simulink model "Assignment2_2017"  (R2017b)
settings: Solver=FixedStepAuto  StartTime=0.0  StopTime=inf  FixedStep=1E-3  RelTol=1e-3  EnableMultiTasking=on
undefined symbols (not defined in the file): D0, D1, D10, D11, D12, D13, D2, D5, D8, D9, PTA0, PTA2, PTB9, PTC16, PTC17, PTC4, PTD0, PTD1, PTD2, PTD3
libraries: frdmk64flib x13, dspswit3 x2
settings Model: ExtModeTrigDuration=5  Creator=Hassan  LastModifiedBy=Hassan
settings OptimizationCC: EnhancedBackFolding=on  PassReuseOutputArgsAs=Individual arguments  MaxStackSize=64  OptimizeBlockOrder=speed  DifferentSizesBufferReuse=on
settings DebuggingCC: ParameterTunabilityLossMsg=error
settings HardwareCC: ProdBitPerPointer=32  ProdBitPerSizeT=32  ProdBitPerPtrDiffT=32  ProdLargestAtomicInteger=Long  ProdLargestAtomicFloat=Double  ProdWordSize=32  ProdHWDeviceType=ARM Compatible->ARM Cortex  UseEmbeddedCoderFeatures=off
settings SFSimCC: SimUseLocalCustomCode=on  MATLABDynamicMemAlloc=off
settings RTWCC: SystemTargetFile=ert.tlc  HardwareBoard=NXP FRDM-K64F  TemplateMakefile=ert_default_tmf  GenerateReport=on  RTWUseLocalCustomCode=on  Toolchain=GNU Tools for ARM Embedded Processors  IncludeHyperlinkInReport=on  LaunchReport=on  GenerateTraceInfo=on  GenerateTraceReport=on  GenerateTraceReportSl=on  GenerateTraceReportSf=on  GenerateTraceReportEml=on
settings CodeAppCC: ForceParamTrailComments=on  IgnoreCustomStorageClasses=off  OperatorAnnotations=on  SimulinkDataObjDesc=on  SFDataObjDesc=on  InsertBlockDesc=on
settings ERTTargetCC: SupportNonInlinedSFcns=on

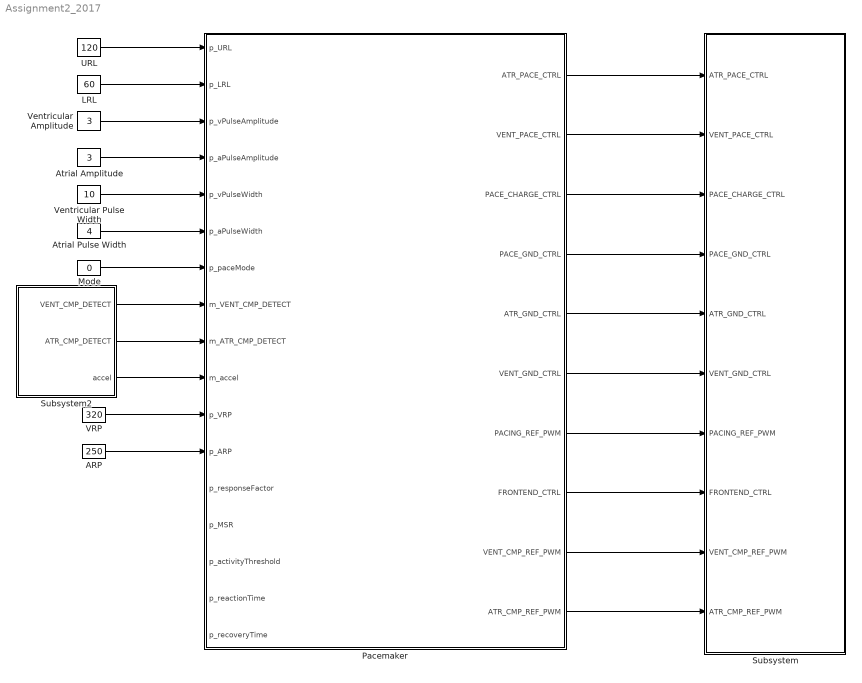
== system Assignment2_2017 ==
  ARP : Constant  Value=250  OutDataTypeStr=double
  Atrial Amplitude : Constant  Value=3  OutDataTypeStr=double
  Atrial Pulse Width : Constant  Value=4  OutDataTypeStr=double
  LRL : Constant  Value=60  OutDataTypeStr=double
  Mode : Constant  Value=0  OutDataTypeStr=uint8
  Pacemaker : Stateflow chart  TreatAsAtomicUnit=on
  Subsystem : Subsystem
  Subsystem2 : Subsystem
  URL : Constant  Value=120  OutDataTypeStr=double
  VRP : Constant  Value=320  OutDataTypeStr=double
  Ventricular Amplitude : Constant  Value=3  OutDataTypeStr=double
  Ventricular Pulse Width : Constant  Value=10  OutDataTypeStr=double
  wires:
  Ventricular Pulse Width/1 -> Pacemaker/5(p_vPulseWidth)
  Mode/1 -> Pacemaker/7(p_paceMode)
  Atrial Pulse Width/1 -> Pacemaker/6(p_aPulseWidth)
  Ventricular Amplitude/1 -> Pacemaker/3(p_vPulseAmplitude)
  LRL/1 -> Pacemaker/2(p_LRL)
  URL/1 -> Pacemaker/1(p_URL)
  Atrial Amplitude/1 -> Pacemaker/4(p_aPulseAmplitude)
  Pacemaker/1(ATR_PACE_CTRL) -> Subsystem/1(ATR_PACE_CTRL)
  Pacemaker/2(VENT_PACE_CTRL) -> Subsystem/2(VENT_PACE_CTRL)
  Pacemaker/3(PACE_CHARGE_CTRL) -> Subsystem/3(PACE_CHARGE_CTRL)
  Pacemaker/4(PACE_GND_CTRL) -> Subsystem/4(PACE_GND_CTRL)
  Pacemaker/5(ATR_GND_CTRL) -> Subsystem/5(ATR_GND_CTRL)
  Pacemaker/6(VENT_GND_CTRL) -> Subsystem/6(VENT_GND_CTRL)
  Pacemaker/7(PACING_REF_PWM) -> Subsystem/7(PACING_REF_PWM)
  Pacemaker/9(VENT_CMP_REF_PWM) -> Subsystem/9(VENT_CMP_REF_PWM)
  Pacemaker/8(FRONTEND_CTRL) -> Subsystem/8(FRONTEND_CTRL)
  Pacemaker/10(ATR_CMP_REF_PWM) -> Subsystem/10(ATR_CMP_REF_PWM)
  VRP/1 -> Pacemaker/11(p_VRP)
  ARP/1 -> Pacemaker/12(p_ARP)
  Subsystem2/1(VENT_CMP_DETECT) -> Pacemaker/8(m_VENT_CMP_DETECT)
  Subsystem2/2(ATR_CMP_DETECT) -> Pacemaker/9(m_ATR_CMP_DETECT)
  Subsystem2/3(accel) -> Pacemaker/10(m_accel)

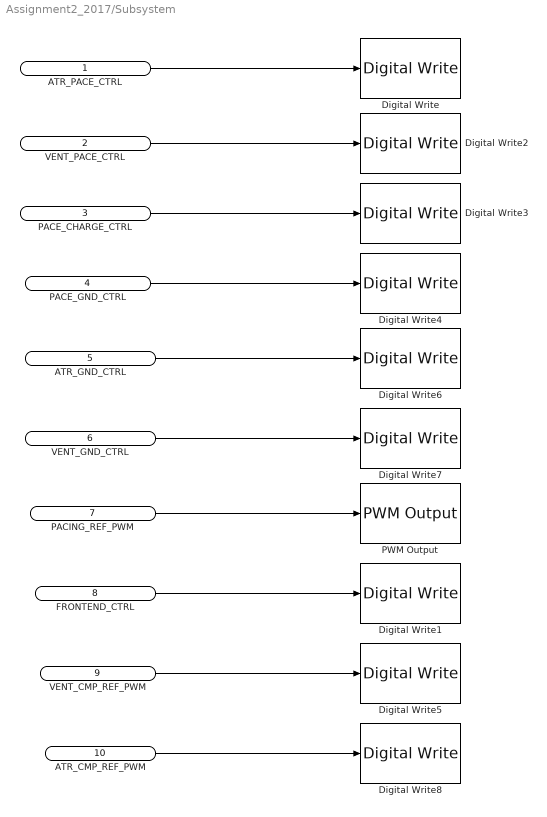
== system Assignment2_2017/Subsystem ==
  ATR_PACE_CTRL : Inport
  VENT_PACE_CTRL : Inport  Port=2
  PACE_CHARGE_CTRL : Inport  Port=3
  PACE_GND_CTRL : Inport  Port=4
  ATR_GND_CTRL : Inport  Port=5
  VENT_GND_CTRL : Inport  Port=6
  PACING_REF_PWM : Inport  Port=7
  FRONTEND_CTRL : Inport  Port=8
  VENT_CMP_REF_PWM : Inport  Port=9
  ATR_CMP_REF_PWM : Inport  Port=10
  Digital Write : frdmk64flib/Digital Write  Whichpin=PTA0 (D8)
      settings: SourceProductName=Simulink Coder Support Package for NXP FRDM-K64F Board
  Digital Write1 : frdmk64flib/Digital Write  Whichpin=PTD1 (D13)
      settings: SourceProductName=Simulink Coder Support Package for NXP FRDM-K64F Board
  Digital Write2 : frdmk64flib/Digital Write  Whichpin=PTC4 (D9)
      settings: SourceProductName=Simulink Coder Support Package for NXP FRDM-K64F Board
  Digital Write3 : frdmk64flib/Digital Write  Whichpin=PTB9 (D2)
      settings: SourceProductName=Simulink Coder Support Package for NXP FRDM-K64F Board
  Digital Write4 : frdmk64flib/Digital Write  Whichpin=PTD0 (D10)
      settings: SourceProductName=Simulink Coder Support Package for NXP FRDM-K64F Board
  Digital Write5 : frdmk64flib/Digital Write  Whichpin=RED_LED
      settings: SourceProductName=Simulink Coder Support Package for NXP FRDM-K64F Board
  Digital Write6 : frdmk64flib/Digital Write  Whichpin=PTD2 (D11)
      settings: SourceProductName=Simulink Coder Support Package for NXP FRDM-K64F Board
  Digital Write7 : frdmk64flib/Digital Write  Whichpin=PTD3 (D12)
      settings: SourceProductName=Simulink Coder Support Package for NXP FRDM-K64F Board
  Digital Write8 : frdmk64flib/Digital Write  Whichpin=RED_LED
      settings: SourceProductName=Simulink Coder Support Package for NXP FRDM-K64F Board
  PWM Output : frdmk64flib/PWM Output  Whichpin=PTA2 (D5)  InitialFrequency=1000  InitialDutyCycle=0
      settings: SourceProductName=Simulink Coder Support Package for NXP FRDM-K64F Board
  wires:
  ATR_PACE_CTRL/1 -> Digital Write/1
  VENT_PACE_CTRL/1 -> Digital Write2/1
  PACE_CHARGE_CTRL/1 -> Digital Write3/1
  PACE_GND_CTRL/1 -> Digital Write4/1
  ATR_GND_CTRL/1 -> Digital Write6/1
  VENT_GND_CTRL/1 -> Digital Write7/1
  PACING_REF_PWM/1 -> PWM Output/1
  FRONTEND_CTRL/1 -> Digital Write1/1
  ATR_CMP_REF_PWM/1 -> Digital Write8/1
  VENT_CMP_REF_PWM/1 -> Digital Write5/1

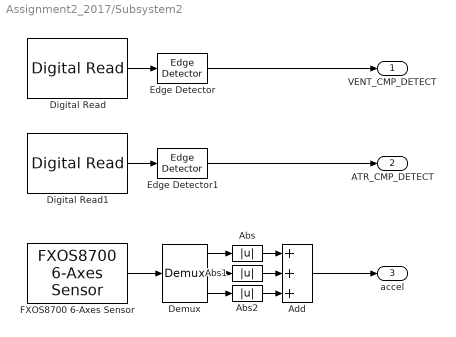
== system Assignment2_2017/Subsystem2 ==
  Abs : Abs
  Abs1 : Abs
  Abs2 : Abs
  Add : Sum  Inputs=+++
  Demux : Demux  Outputs=3
  Digital Read : frdmk64flib/Digital Read  Whichpin=PTC17 (D1)  SampleTime=-1
      settings: SourceProductName=Simulink Coder Support Package for NXP FRDM-K64F Board
  Digital Read1 : frdmk64flib/Digital Read  Whichpin=PTC16 (D0)  SampleTime=-1
      settings: SourceProductName=Simulink Coder Support Package for NXP FRDM-K64F Board
  Edge Detector : dspswit3/Edge Detector
      settings: SourceProductName=DSP System Toolbox  SourceProductBaseCode=DS
  Edge Detector1 : dspswit3/Edge Detector
      settings: SourceProductName=DSP System Toolbox  SourceProductBaseCode=DS
  FXOS8700 6-Axes Sensor : frdmk64flib/FXOS8700 6-Axes Sensor  Activesensor=Accelerometer only  ODR=400Hz  HybridODR=400Hz  Accelfullrange=-4g to +4g  SampleTime=-1
      settings: SourceProductName=Simulink Coder Support Package for NXP FRDM-K64F Board
  VENT_CMP_DETECT : Outport
  ATR_CMP_DETECT : Outport  Port=2
  accel : Outport  Port=3
  wires:
  Digital Read/1 -> Edge Detector/1
  Digital Read1/1 -> Edge Detector1/1
  Edge Detector1/1 -> ATR_CMP_DETECT/1
  Edge Detector/1 -> VENT_CMP_DETECT/1
  FXOS8700 6-Axes Sensor/1 -> Demux/1
  Add/1 -> accel/1
  Demux/1 -> Abs/1
  Abs/1 -> Add/1
  Demux/2 -> Abs1/1
  Abs1/1 -> Add/2
  Demux/3 -> Abs2/1
  Abs2/1 -> Add/3

== stateflow chart Assignment2_2017/Pacemaker ==
  state Init
  state SetPulseRate
    entry:
    VVtime=(60000/p_LRL)-p_vPulseWidth;
    AAtime=(60000/p_LRL)-p_aPulseWidth;
  state VentricleSensingInit
    entry:
    VENT_CMP_REF_PWM = (3.3/3.3)*100;
    FRONTEND_CTRL=1;
  state ModeChange
    entry:
    FRONTEND_CTRL=0;
  state AtriumSensingInit
    entry:
    ATR_CMP_REF_PWM = (3.3/3.3)*100;
    FRONTEND_CTRL=1;
  state ChargeC22DischargeC21
    % Charging C22 and discharging C21
    entry:
    % Charge C22
    VENT_PACE_CTRL=0;
    PACING_REF_PWM=(pulseAmplitude/5.0)*100;
    PACE_CHARGE_CTRL=1;
    %Discharge C21
    PACE_GND_CTRL=1;
    VENT_GND_CTRL=1;
  state PaceAtrium
    %PACE ATRIUM
    entry:
    PACE_CHARGE_CTRL=0;
    PACE_GND_CTRL=1;
    ATR_GND_CTRL=0;
    ATR_PACE_CTRL=1;
  state CheckAccelUpdateRate
    entry:
    updateRate();
  state PaceVentricle
    %PACE VENTRICLE
    entry:
    PACE_CHARGE_CTRL=0;
    PACE_GND_CTRL=1;
    VENT_GND_CTRL=0;
    VENT_PACE_CTRL=1;
  state VRP
  state ARP
  state VentBeatSensed
  state AtrBeatSensed
  (default) -> Init
  Init -> SetPulseRate
  (junction 72) -> VentricleSensingInit [order 1] : [p_paceMode==4 || p_paceMode==5]
  SetPulseRate -> (junction 72) [order 1] : [p_paceMode>=4]
  ModeChange -> SetPulseRate
  (junction 72) -> AtriumSensingInit [order 2] : [p_paceMode==6 || p_paceMode==7]
  VentricleSensingInit -> (junction 84)
  SetPulseRate -> ChargeC22DischargeC21 [order 2] : [p_paceMode<4]
  AtriumSensingInit -> (junction 84)
  (junction 84) -> ChargeC22DischargeC21
  (junction 144) -> ModeChange [order 2]
  ChargeC22DischargeC21 -> PaceAtrium [order 4] : [(p_paceMode==2 || p_paceMode==3) && after(AAtime, msec)]
  PaceAtrium -> (junction 144) : [after(p_aPulseWidth,msec)]
  CheckAccelUpdateRate -> ModeChange
  PaceVentricle -> (junction 144) : [after(p_vPulseWidth,msec)]
  (junction 144) -> CheckAccelUpdateRate [order 1] : [p_paceMode==1 || p_paceMode==3]
  ChargeC22DischargeC21 -> PaceVentricle [order 3] : [(p_paceMode==0 || p_paceMode==1) && after(VVtime, msec)]
  ChargeC22DischargeC21 -> VentBeatSensed [order 2] : [m_VENT_CMP_DETECT == 1]
  VRP -> ChargeC22DischargeC21 : [after(p_VRP,msec)]
  ARP -> ChargeC22DischargeC21 : [after(p_ARP,msec)]
  ChargeC22DischargeC21 -> AtrBeatSensed [order 1] : [m_ATR_CMP_DETECT==1]
  VentBeatSensed -> VRP
  AtrBeatSensed -> ARP
  data: p_URL input double; p_LRL input double; p_vPulseAmplitude input double; ATR_PACE_CTRL output uint16; VENT_PACE_CTRL output uint16; PACE_CHARGE_CTRL output uint16; PACE_GND_CTRL output uint16; ATR_GND_CTRL output uint16; VENT_GND_CTRL output uint16; p_aPulseAmplitude input double; p_vPulseWidth input double; p_aPulseWidth input double; p_paceMode input uint8; PACING_REF_PWM output double; FRONTEND_CTRL output uint16; VENT_CMP_REF_PWM output double; ATR_CMP_REF_PWM output double; m_VENT_CMP_DETECT input double; m_ATR_CMP_DETECT input double; m_accel input double; p_VRP input double; p_ARP input double; p_responseFactor input uint8; p_MSR input double; p_activityThreshold input uint8; p_reactionTime input double; p_recoveryTime input double; VVtime local double; AAtime local double
  function updateRate:
    | function updateRate()
    | 
    | if (m_accel>=p_activityThreshold)
    | 
    | end
